simulink model "untitled"  (R2015a)
settings: Solver=ode45  StartTime=0.0  StopTime=40  RelTol=1e-3
libraries: cstblocks x1, simulink x1
settings Model: Creator=saadc  LastModifiedBy=saadc

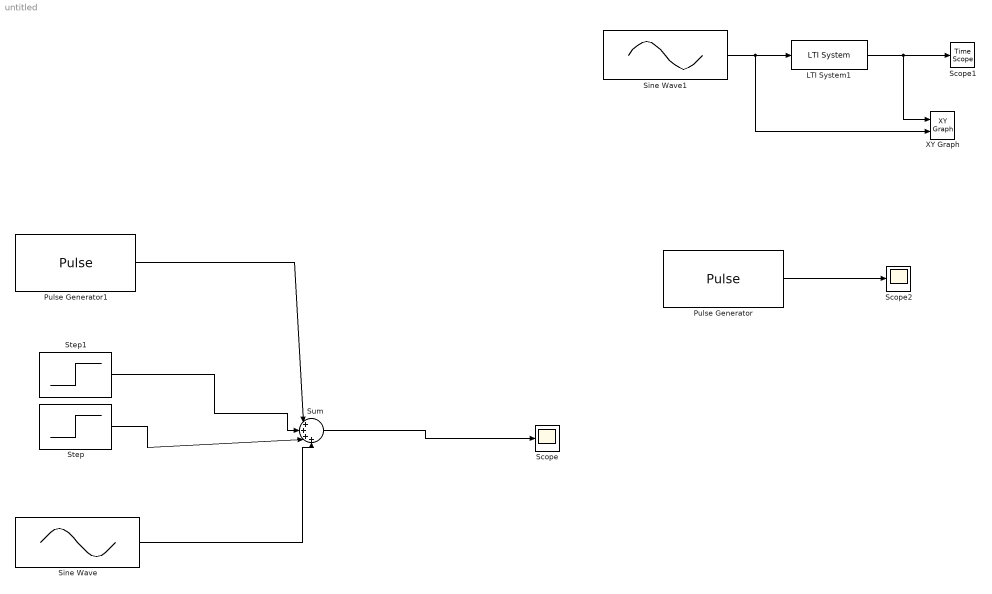
== system untitled ==
  LTI System1 : cstblocks/LTI System  sys=tf(10,[1 2 20])  IC=[]
  Pulse Generator : DiscretePulseGenerator  PulseType=Time based  Period=10  PulseWidth=5
  Pulse Generator1 : DiscretePulseGenerator  PulseType=Time based  Period=10  PulseWidth=5
  Scope : Scope
  Scope1 : TimeScope
  Scope2 : Scope
      settings: SaveName=ScopeData2
  Sine Wave : Sin  SampleTime=0
  Sine Wave1 : Sin  SampleTime=0
  Step : Step  Time=2  After=4  SampleTime=0
  Step1 : Step  Time=2  After=4  SampleTime=0
  Sum : Sum  Inputs=|++++
  XY Graph : simulink/Sinks/XY Graph  xmin=-1  xmax=1  ymin=-1  ymax=1  st=-1
  wires:
  Sine Wave/1 -> Sum/4
  Sum/1 -> Scope/1
  Step/1 -> Sum/3
  Step1/1 -> Sum/2
  Sine Wave1/1 -> XY Graph/2, LTI System1/1
  LTI System1/1 -> XY Graph/1, Scope1/1
  Pulse Generator/1 -> Scope2/1
  Pulse Generator1/1 -> Sum/1
